simulink library "dhp"  (R2021b)
settings: Solver=VariableStepAuto  StartTime=0.0  StopTime=10.0  RelTol=1e-3
undefined symbols (not defined in the file or in its folder): ADHP_HysOffset_X_pct, ENUM_POWERSTA_OFF, ENUM_POWERSTA_STANDBY, ENUM_RANGESTA_12IN, ENUM_RANGESTA_12OUT, ENUM_RANGESTA_1OUT, ENUM_RANGESTA_2OUT, ENUM_RESETPEDALZEROPOSREQ_START, FALSE, HUNDRED, KDHP_AcceleratorLoadScalr_gain, KDHP_AccPedalDepressed_pct, KDHP_AccPedalReleased_pct, KDHP_ActAPSPosn_pct_ovrdflg, KDHP_ActAPSPosn_pct_ovrdval, KDHP_DeadBand_pct, KDHP_EAPS11OutWT_gain, KDHP_EAPS12Disagree_pct, KDHP_EAPS12DisagreeTime_s, KDHP_EAPS12OutWT_gain, KDHP_EAPS1AOutWT_gain, KDHP_EAPS1BADHigh_pct, KDHP_EAPS1BADLow_pct, KDHP_EAPS1BADTime_s, KDHP_EAPS1Min_pct_ovrdflg, KDHP_EAPS1Min_pct_ovrdval, KDHP_EAPS1MINInitLowLim_pct, KDHP_EAPS1MINInitUpLim_pct, KDHP_EAPS1WT_gain, KDHP_EAPS21OutWT_gain, KDHP_EAPS22OutWT_gain, KDHP_EAPS2AOutWT_gain, KDHP_EAPS2BADHigh_pct, KDHP_EAPS2BADLow_pct, KDHP_EAPS2BADTime_s, KDHP_EAPS2Min_pct_ovrdflg, KDHP_EAPS2Min_pct_ovrdval, KDHP_EAPS2MINInitLowLim_pct, KDHP_EAPS2MINInitUpLim_pct, KDHP_EAPS2Offset_pct, KDHP_EAPS2Scaler_gain, KDHP_EAPS2WT_gain, KDHP_EAPSCRBadWDSP_pct, KDHP_EAPSLearnDwHigh_pct, KDHP_EAPSLearnDwLow_pct, KDHP_EAPSLearnDwMAX_pct, KDHP_EAPSLearnUpHigh_pct, KDHP_EAPSLearnUpLow_pct, KDHP_EAPSLearnUpOffset_pct, KDHP_EAPSMINLowerLimit_pct, KDHP_EAPSStableThrsh_pct, KDHP_EAPSStableTime_s, KDHP_EPEDPOSNUpLimit_pct, KDHP_GetNRMBaseTime_s, KDHP_LVBattHigh_V, KDHP_LVBattHighLimit_V, KDHP_LVBattLow_V, MDHP_HysOffset_Y_pct, TRUE, ZERO_FLOAT
libraries: hcu_lib x6, simulink x4
(part 2 of 2)

== stateflow chart dhp/DHP/DHP/APS_calaulation/Calculation/Chart ==
  state PedalIncreasing
    en:
    VDHP_PedalIncreasing_flg = TRUE;
    VDHP_Inc2Dec_flg = FALSE;
    VDHP_EPEDLINDMem_pct = VDHP_EPEDLIND_pct;
    state PctMemorize
      en:
      VDHP_Inc2DecPctMemorize_flg = FALSE;
      (default) -> (junction 12)
      PedalIncreasing.PctMemorize -> (junction 12) [order 1]
      (junction 12) -> (junction 14) [order 1] : [VDHP_EPEDLIND_pct  > KDHP_DeadBand_pct &&...
          | (VDHP_EPEDLIND_pct - VDHP_EPEDLINDLast_pct) < ZERO_FLOAT]
      (junction 12) -> (junction 18) [order 2]
      (junction 14) -> (junction 16) : {
          | VDHP_Inc2DecPctMemorize_flg = TRUE;
          | }
      (junction 16) -> (junction 18)
    state Judgement
      (default) -> (junction 22) : {
          | VDHP_EPEDLINDMem_pct = VDHP_EPEDLIND_pct;
          | VDHP_Inc2DecMemoryReset_flg = FALSE;
          | }
      PedalIncreasing.Judgement -> (junction 22) [order 1]
      (junction 22) -> (junction 24) [order 1] : [(VDHP_EPEDLINDMem_pct - VDHP_EPEDLIND_pct ) > VDHP_HysOffset_pct]
      (junction 22) -> (junction 28) [order 2]
      (junction 24) -> (junction 26) : {
          | VDHP_Inc2Dec_flg = TRUE;
          | }
      (junction 28) -> (junction 30) [order 1] : [(VDHP_EPEDLINDMem_pct - VDHP_EPEDLIND_pct) < ZERO_FLOAT]
      (junction 28) -> (junction 36) [order 2]
      (junction 30) -> (junction 32) : {
          | VDHP_Inc2DecMemoryReset_flg = TRUE;
          | }
      (junction 32) -> (junction 36)
      (junction 26) -> (junction 32)
    (default) -> PedalIncreasing.PctMemorize
    PedalIncreasing.PctMemorize -> PedalIncreasing.Judgement [order 1] : [VDHP_Inc2DecPctMemorize_flg]
    PedalIncreasing.Judgement -> PedalIncreasing.PctMemorize [order 1] : [VDHP_Inc2DecMemoryReset_flg ||...
        | (VDHP_EPEDLIND_pct  < KDHP_DeadBand_pct)]
  state PedalDecreasing
    en:
    VDHP_PedalIncreasing_flg = FALSE;
    VDHP_Dec2Inc_flg = FALSE;
    state PctMemorize
      en:
      VDHP_Dec2IncPctMemorize_flg = FALSE;
      (default) -> (junction 46)
      PedalDecreasing.PctMemorize -> (junction 46) [order 1]
      (junction 46) -> (junction 47) [order 1] : [(VDHP_EPEDLIND_pct - VDHP_EPEDLINDLast_pct) > ZERO_FLOAT]
      (junction 46) -> (junction 48) [order 2]
      (junction 47) -> (junction 49) : {
          | VDHP_Dec2IncPctMemorize_flg = TRUE;
          | }
      (junction 49) -> (junction 48)
    state Judgement
      (default) -> (junction 58) : {
          | VDHP_EPEDLINDMem_pct = VDHP_EPEDLIND_pct;
          | VDHP_Dec2IncMemoryReset_flg = FALSE;
          | }
      PedalDecreasing.Judgement -> (junction 58) [order 1]
      (junction 58) -> (junction 59) [order 1] : [(VDHP_EPEDLIND_pct - VDHP_EPEDLINDMem_pct) > VDHP_HysOffset_pct]
      (junction 58) -> (junction 60) [order 2]
      (junction 59) -> (junction 64) : {
          | VDHP_Dec2Inc_flg = TRUE;
          | }
      (junction 60) -> (junction 61) [order 1] : [VDHP_EPEDLINDMem_pct - VDHP_EPEDLIND_pct > ZERO_FLOAT]
      (junction 60) -> (junction 62) [order 2]
      (junction 61) -> (junction 63) : {
          | VDHP_Dec2IncMemoryReset_flg = TRUE;
          | }
      (junction 63) -> (junction 62)
      (junction 64) -> (junction 63)
    (default) -> PedalDecreasing.PctMemorize
    PedalDecreasing.PctMemorize -> PedalDecreasing.Judgement [order 1] : [VDHP_Dec2IncPctMemorize_flg]
    PedalDecreasing.Judgement -> PedalDecreasing.PctMemorize [order 1] : [VDHP_Dec2IncMemoryReset_flg]
  (default) -> PedalIncreasing
  PedalIncreasing -> PedalDecreasing : [VDHP_Inc2Dec_flg]
  PedalDecreasing -> PedalIncreasing : [VDHP_Dec2Inc_flg || (VDHP_EPEDLIND_pct  < KDHP_DeadBand_pct)]
  data: KDHP_DeadBand_pct input; VDHP_EPEDLINDLast_pct input; VDHP_EPEDLIND_pct input; VDHP_HysOffset_pct input; VDHP_PedalIncreasing_flg output boolean; VDHP_Dec2IncMemoryReset_flg local boolean; VDHP_Dec2IncPctMemorize_flg local boolean; VDHP_Dec2Inc_flg local boolean; VDHP_EPEDLINDMem_pct local double; VDHP_Inc2DecMemoryReset_flg local boolean; VDHP_Inc2DecPctMemorize_flg local boolean; VDHP_Inc2Dec_flg local boolean; FALSE parameter; TRUE parameter; ZERO_FLOAT parameter
